simulink model "TVLQR_w_pss"  (R2024b)
settings: Solver=FixedStepDiscrete  StartTime=0.0  StopTime=11380*10  FixedStep=1  RelTol=1e-3
values from neighbouring files (symbols this model uses):
  Ad = sys_d.A    [TVLQR2.m]    (also in TVLQR_dist.m)
  Bd = sys_d.B    [TVLQR2.m]    (also in TVLQR_dist.m)
  Cd = sys_d.C    [TVLQR2.m]    (also in TVLQR_dist.m)
  Dd = sys_d.D    [TVLQR2.m]    (also in TVLQR_dist.m)
  dt_sim = 0.1    [TVLQR2.m]    (also in TVLQR_dist.m)
  K_tv = zeros(3,6,N_orbit)    [TVLQR2.m]    (also in TVLQR_dist.m)
  m_max_pss = 0.166    [TVLQR2.m]    (also in TVLQR_dist.m)
  N_orbit = round(T_total / dt_sim)    [TVLQR2.m]    (also in TVLQR_dist.m)
  T_total = length(t_trim)*dt_data    [Bdot_run.m]    (also in TVLQR2.m = length(t_tv_trimmed) * dt_data; TVLQR_dist.m = length(t_tv_trimmed) * dt_data)
settings Model: Creator=zalak  LastModifiedBy=zalak

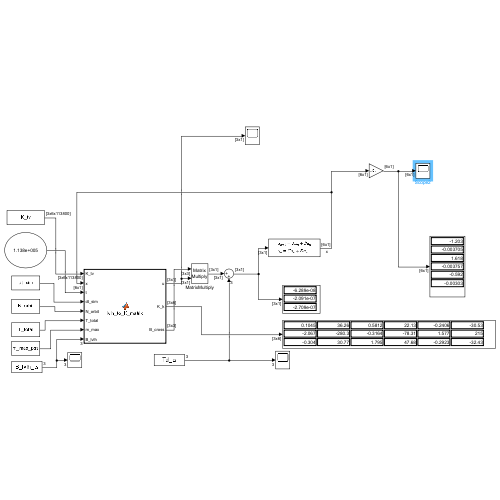
[thumbnail: Simulink's stored preview of the top-level diagram]
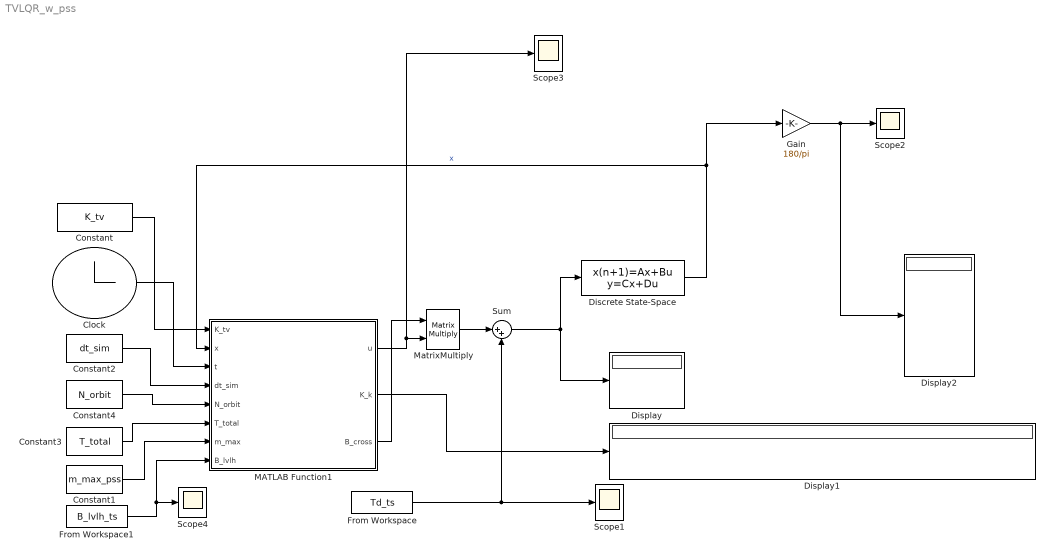
== system TVLQR_w_pss ==
  Clock : Clock
  Constant : Constant  Value=K_tv
  Constant1 : Constant  Value=m_max_pss
  Constant2 : Constant  Value=dt_sim
  Constant3 : Constant  Value=T_total
  Constant4 : Constant  Value=N_orbit
  Discrete State-Space : DiscreteStateSpace  A=Ad  B=Bd  C=Cd  D=Dd  InitialCondition=[20*pi/180;0;0;0;0;0]
  Display : Display
  Display1 : Display
  Display2 : Display
  From Workspace : FromWorkspace  VariableName=Td_ts
  From Workspace1 : FromWorkspace  VariableName=B_lvlh_ts  SampleTime=1
  Gain : Gain  Gain=180/pi
  MATLAB Function1 : MATLAB Function  TreatAsAtomicUnit=on
  MatrixMultiply : Product  Multiplication=Matrix(*)
  Scope{1..4} (4 alike) : Scope
  Sum : Sum  Inputs=|++
  wires:
  Gain/1 -> Display2/1, Scope2/1
  From Workspace1/1 -> MATLAB Function1/8(B_lvlh), Scope4/1
  Constant2/1 -> MATLAB Function1/4(dt_sim)
  MATLAB Function1/1(u) -> Scope3/1, MatrixMultiply/2
  Discrete State-Space/1 -> Gain/1, MATLAB Function1/2(x)  "x"
  MATLAB Function1/3(B_cross) -> MatrixMultiply/1
  MatrixMultiply/1 -> Sum/1
  From Workspace/1 -> Sum/2, Scope1/1
  Sum/1 -> Discrete State-Space/1, Display/1
  Constant/1 -> MATLAB Function1/1(K_tv)
  Constant1/1 -> MATLAB Function1/7(m_max)
  Constant3/1 -> MATLAB Function1/6(T_total)
  Constant4/1 -> MATLAB Function1/5(N_orbit)
  Clock/1 -> MATLAB Function1/3(t)
  MATLAB Function1/2(K_k) -> Display1/1

== matlab function TVLQR_w_pss/MATLAB Function1 ==
  data: K_tv input; x input; t input; dt_sim input; N_orbit input; T_total input; m_max input; B_lvlh input; u output; K_k output; B_cross output
function [u, K_k, B_cross] = lvlh_to_K_matrix(K_tv, x, t, dt_sim, N_orbit, T_total, m_max, B_lvlh)
% TVLQR step — dipole-based magnetorquer control
%
%   u (3x1)   commanded magnetic dipole moment [A·m²]
%   K (3x6)   instantaneous LQR gain
%   P_next    Riccati state to feed back next step
%
% State convention (matches the A used in setup):
%   x = [phi, p, psi, r, theta, q]'
%       roll, roll-rate, yaw, yaw-rate, pitch, pitch-rate
% GOOSE 2U inertia [kg·m²]

%% Step 1 —  Find Magnetic field Cross product (B_cross)
Bx = B_lvlh(1);  By = B_lvlh(2);  Bz = B_lvlh(3);
B_cross = [   0,   Bz,  -By;
            -Bz,    0,   Bx;
             By,  -Bx,    0 ];

%% Step 2: Find current index in the periodic schedule
t_mod = mod(t, T_total);
k = floor(t_mod / dt_sim) + 1;
k = min(max(k, 1), N_orbit);

K_k = K_tv(:,:,k);
u_nom = -K_k * x;

if t == 1
    disp(K_k)
end

% Saturate (Psiaki proportional)
beta = max(abs(u_nom) / m_max);
if beta <= 1
    u = u_nom;
else
    u = u_nom / beta;
end
end
